simulink model "task_5"  (Simulink 7.6)
settings: Solver=ode45  StartTime=3  StopTime=10  RelTol=1e-3
libraries: simulink x1
settings Model: Creator=Admin  LastModifiedBy=Admin

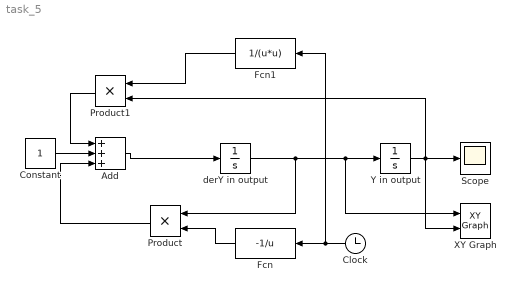
== system task_5 ==
  Add : Sum  Inputs=+++
  Clock : Clock
      settings: Decimation=10
  Constant : Constant
  Fcn : Fcn  Expr=-1/u
  Fcn1 : Fcn  Expr=1/(u*u)
  Product : Product  RndMeth=Zero
  Product1 : Product  RndMeth=Zero
  Scope : Scope
  XY Graph : simulink/Sinks/XY Graph  SystemSampleTime=-1  xmin=3  xmax=8  ymin=0  ymax=40  st=-1
  Y in output : Integrator  InitialCondition=6
  derY in output : Integrator  InitialCondition=3
  wires:
  derY in output/1 -> Product/1, Y in output/1, XY Graph/1
  Clock/1 -> Fcn/1, Fcn1/1
  Fcn/1 -> Product/2
  Add/1 -> derY in output/1
  Product/1 -> Add/3
  Constant/1 -> Add/2
  Product1/1 -> Add/1
  Fcn1/1 -> Product1/1
  Y in output/1 -> Product1/2, Scope/1, XY Graph/2
